simulink model "Car_like_robot_trajectory_tracking"  (R2018a)
settings: Solver=ode4  StartTime=0.0  StopTime=63  FixedStep=Ts  RelTol=1e-3
values from neighbouring files (symbols this model uses):
  Delta = 0.35    [Invariant_set_Trajectory_Tracking_Control_approachACC23.m]    (also in Simulink_model_parameters.m)
  l = 0.5    [Invariant_set_Trajectory_Tracking_Control_approachACC23.m]    (also in Simulink_model_parameters.m = 0.256)
  phi0 = phir(1)    [Invariant_set_Trajectory_Tracking_Control_approachACC23.m]    (also in Simulink_model_parameters.m = 0)
  theta0 = thetar(1)    [Invariant_set_Trajectory_Tracking_Control_approachACC23.m]    (also in Simulink_model_parameters.m)
  x0 = 0    [Invariant_set_Trajectory_Tracking_Control_approachACC23.m]    (also in Simulink_model_parameters.m = xr(1))
  y0 = -0.035    [Invariant_set_Trajectory_Tracking_Control_approachACC23.m]    (also in Simulink_model_parameters.m = yr(1))
undefined symbols (not defined in the file or in its folder): K_LQ
libraries: simulink x2
settings Model: Creator=cricr  LastModifiedBy=cricr

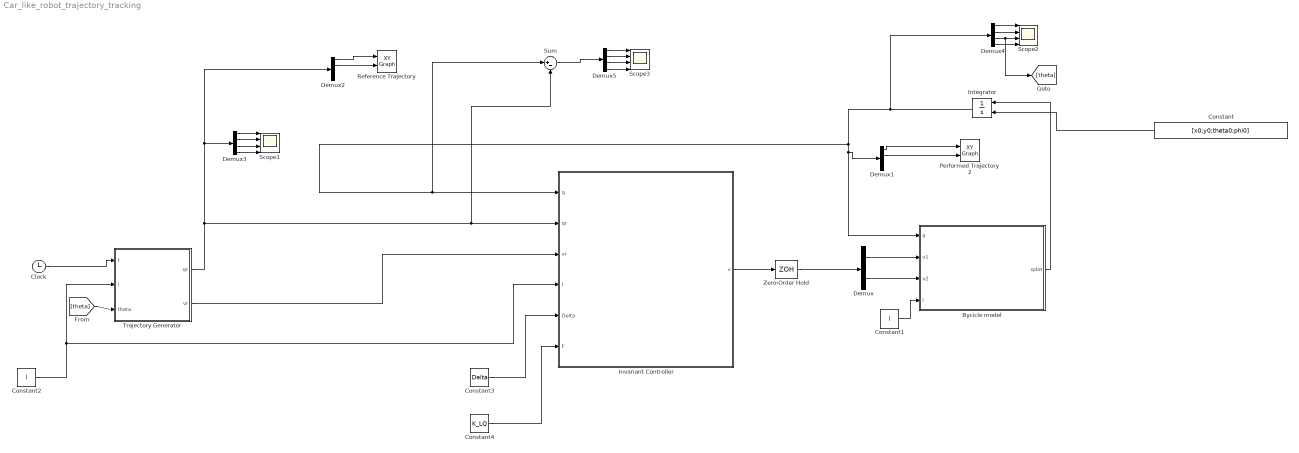
== system Car_like_robot_trajectory_tracking ==
  "Bycicle model " : MATLAB Function  TreatAsAtomicUnit=on
  Clock : Clock
  Constant : Constant  Value=[x0;y0;theta0;phi0]
  Constant1 : Constant  Value=l
  Constant2 : Constant  Value=l
  Constant3 : Constant  Value=Delta
  Constant4 : Constant  Value=K_LQ
  Demux : Demux  Outputs=2
  Demux{1..5} (5 alike) : Demux
  Integrator : Integrator  InitialConditionSource=external
  Invariant Controller : MATLAB Function  TreatAsAtomicUnit=on
  Performed Trajectory 2 : simulink/Sinks/XY Graph  xmin=-3  xmax=3  ymin=-3  ymax=3  st=Ts
  Reference Trajectory : simulink/Sinks/XY Graph  xmin=-3  xmax=3  ymin=-3  ymax=3  st=Ts
  Scope1 : Scope  NumInputPorts=4
  Scope2 : Scope  NumInputPorts=4
  Scope3 : Scope  NumInputPorts=4
  Sum : Sum  Inputs=|+-
  Trajectory Generator : MATLAB Function  TreatAsAtomicUnit=on
  Zero-Order Hold : ZeroOrderHold  SampleTime=-1
  wires:
  Constant/1 -> Integrator/2
  Integrator/1 -> Demux4/1, Demux1/1, "Bycicle model "/1(q), Sum/1, Invariant Controller/1(q)
  Constant1/1 -> "Bycicle model "/4(l)
  Clock/1 -> Trajectory Generator/1(t)
  Trajectory Generator/1(qr) -> Sum/2, Invariant Controller/2(qr), Demux3/1, Demux2/1
  Trajectory Generator/2(vr) -> Invariant Controller/3(vr)
  Constant2/1 -> Trajectory Generator/2(l), Invariant Controller/4(l)
  Constant3/1 -> Invariant Controller/5(Delta)
  Invariant Controller/1(v) -> Zero-Order Hold/1
  Constant4/1 -> Invariant Controller/6(F)
  Demux2/1 -> Reference Trajectory/1
  Demux2/2 -> Reference Trajectory/2
  Demux3/1 -> Scope1/1
  Demux3/2 -> Scope1/2
  Demux3/3 -> Scope1/3
  Demux3/4 -> Scope1/4
  Demux/1 -> "Bycicle model "/2(v1)
  Demux/2 -> "Bycicle model "/3(v2)
  Demux1/1 -> Performed Trajectory 2/1
  Demux1/2 -> Performed Trajectory 2/2
  Demux4/4 -> Scope2/4
  Demux4/2 -> Scope2/2
  Demux4/3 -> [theta], Scope2/3
  Demux4/1 -> Scope2/1
  Demux5/2 -> Scope3/2
  Demux5/4 -> Scope3/4
  Demux5/1 -> Scope3/1
  Demux5/3 -> Scope3/3
  Sum/1 -> Demux5/1
  Zero-Order Hold/1 -> Demux/1
  [theta] -> Trajectory Generator/3(theta)
  "Bycicle model "/1(qdot) -> Integrator/1

== matlab function Car_like_robot_trajectory_tracking/Invariant Controller ==
  data: q input; v output; qr input; vr input; l input; Delta input; F input
function v = tracking_controller(q,qr,vr,l,Delta,F)
x=q(1); y=q(2); theta=q(3); phi=q(4);
xr=qr(1); yr=qr(2); thetar=qr(3); phir=qr(4);
v1r=vr(1); v2r=vr(2);


%Feedback linearized system state
z_k=[x+l*cos(theta)+Delta*cos(phi+theta);
     y+l*sin(theta)+Delta*sin(phi+theta)];
 
%Feedback linearized system reference trajectory
zr_k=[xr+l*cos(thetar)+Delta*cos(phir+thetar);
      yr+l*sin(thetar)+Delta*sin(phir+thetar)];


%Feedback Linearization state transformation
T_FL=[cos(theta)-tan(phi)*(sin(theta)+Delta*sin(theta+phi)/l) -Delta*sin(theta+phi); 
      sin(theta)+tan(phi)*(cos(theta)+Delta*cos(theta+phi)/l) Delta*cos(theta+phi)];

%Feedback Linearization reference transformation
T_FL_r=[cos(thetar)-tan(phir)*(sin(thetar)+Delta*sin(thetar+phir)/l) -Delta*sin(thetar+phir);
     sin(thetar)+tan(phir)*(cos(thetar)+Delta*cos(thetar+phir)/l) Delta*cos(thetar+phir)];
 
ur=T_FL_r*[v1r;v2r];


%Error Trajectory 
z_tilde=z_k-zr_k;


%Linear control law 
uk=-F*z_tilde+ur;

v=inv(T_FL)*uk;

== matlab function Car_like_robot_trajectory_tracking/Bycicle model  ==
  data: q input; qdot output; v1 input; v2 input; l input
function qdot  = bycicle_model(q,v1,v2,l)

%This function implements the car kinematic model
x=q(1);
y=q(2);
theta=q(3);
phi=q(4);

q1dot=v1*cos(theta);
q2dot=v1*sin(theta);
q3dot = v1*tan(phi)/l;
q4dot = v2;


qdot= [q1dot;q2dot;q3dot;q4dot];
end

== matlab function Car_like_robot_trajectory_tracking/Trajectory Generator ==
  data: t input; qr output; vr output; l input; theta input
function [qr, vr] = Trajectory(t,l,theta)

vxbar=2; vybar=2; alpha=10;

xr=vxbar*cos(t/alpha)-(l/2)*cos(theta);
yr=vybar*sin(t/alpha)-(l/2)*sin(theta);

xdr=-1/alpha*vxbar*sin(t/alpha);
ydr= 1/alpha*vybar*cos(t/alpha);

xddr=-1/alpha^2*vxbar*cos(t/alpha);
yddr=-1/alpha^2*vybar*sin(t/alpha);

xdddr=1/alpha^3*vxbar*sin(t/alpha);
ydddr=-1/alpha^3*vybar*cos(t/alpha);



%Driving velocity reference
v1r=sqrt(xdr^2+ydr^2); %Linear velocity of the trajectory


%Trajectory Orientation
if t<15.8
    thetar=atan2(ydr/v1r,xdr/v1r); 
else
thetar=atan2(ydr/v1r,xdr/v1r)+2*pi;
end




%Vehicle Angular velocity reference
thetadr=(yddr*xdr-xddr*ydr)/v1r^2; %Angular velocity velocity of the trajectory

%Steering angle reference
phir=atan(l*(yddr*xdr-xddr*ydr)/v1r^3);

%Steering velocity reference
v2r=l*v1r*((ydddr*xdr-xdddr*ydr)*v1r^2-3*(yddr*xdr-xddr*ydr)*(xdr*xddr+ydr*yddr))/(v1r^6+l^2*(yddr*xdr-xddr*ydr)^2);


%Nonlinear model reference state
qr=[xr;yr;thetar;phir];
vr=[v1r;v2r];
